simulink model "model_dyskretny_2_for_print"  (R2020a)
settings: Solver=VariableStepAuto  StartTime=0.0  StopTime=10.0  RelTol=1e-3
values from neighbouring files (symbols this model uses):
  T = 0.5    [pom.m]    (also in zad1_10.m; zad1_4.m; zad1_6_1.m; zad1_6_2.m)
settings Model: Creator=jakub  LastModifiedBy=jakub

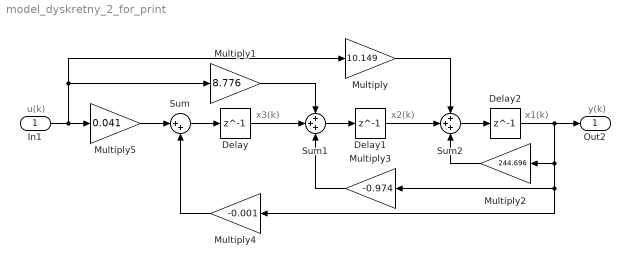
== system model_dyskretny_2_for_print ==
  note: y(k)
  note: u(k)
  note: x2(k)
  note: x3(k)
  note: x1(k)
  In1 : Inport
  Delay : Delay  DelayLength=1  InitialCondition=0  SampleTime=T
  Delay1 : Delay  DelayLength=1  InitialCondition=0  SampleTime=T
  Delay2 : Delay  DelayLength=1  InitialCondition=0  SampleTime=T
  Multiply : Gain  Gain=10.149
  Multiply1 : Gain  Gain=8.776
  Multiply2 : Gain  Gain=244.696
  Multiply3 : Gain  Gain=-0.974
  Multiply4 : Gain  Gain=-0.001
  Multiply5 : Gain  Gain=0.041
  Sum : Sum  Inputs=|++
  Sum1 : Sum  Inputs=+++
  Sum2 : Sum  Inputs=+++
  Out2 : Outport
  wires:
  In1/1 -> Multiply5/1, Multiply/1, Multiply1/1
  Sum/1 -> Delay/1
  Multiply5/1 -> Sum/1
  Sum1/1 -> Delay1/1
  Delay1/1 -> Sum2/2
  Sum2/1 -> Delay2/1
  Delay/1 -> Sum1/2
  Delay2/1 -> Multiply4/1, Multiply3/1, Multiply2/1, Out2/1
  Multiply1/1 -> Sum1/1
  Multiply/1 -> Sum2/1
  Multiply3/1 -> Sum1/3
  Multiply4/1 -> Sum/2
  Multiply2/1 -> Sum2/3
